simulink model "dqpsk_plot"  (Simulink 4.00)
settings: Solver=ode45  StartTime=0.0  StopTime=10.0  RelTol=1e-3
undefined symbols (not defined in the file): slcm
libraries: commdigbbndpm2 x1, commsource2 x1, simulink3 x1
settings Model: LastModifiedBy=agaltman  BlockReductionOpt=off

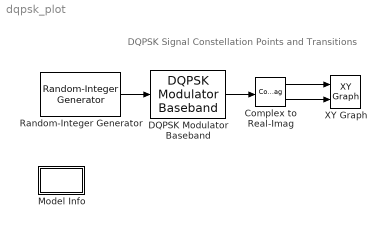
== system dqpsk_plot ==
  note: DQPSK Signal Constellation Points and Transitions
  Complex to Real-Imag : ComplexToRealImag  Output=RealAndImag
  DQPSK Modulator Baseband : commdigbbndpm2/DQPSK Modulator Baseband  InType=Integer  Enc=Binary  Ph=pi/4  numSamp=1
  Model Info : Subsystem  LoadFcn=slcm LoadBlock;  InitFcn=slcm('UpdateAllCMBlocksInThisModelInit')  mask(CMBlock){InitialSaveTempField=, InitialBlockCM=none, BlockCM=none, Frame=on, SaveTempField=, DisplayStringWithTags=Info, MaskDisplayString=Info, HorizontalTextAlignment=Center, LeftAlignmentValue=0.5, SourceBlockDiagram=dqpsk_plot, TagMaxNumber=20, CMTag1=, CMTag2=, CMTag3=, CMTag4=, CMTag5=, CMTag6=, CMTag7=, CMTag8=, CMTag9=, CMTag10=, CMTag11=, CMTag12=, CMTag13=, CMTag14=, CMTag15=, CMTag16=, CMTag17=, CMTag18=, CMTag19=, CMTag20=}
      mask help: This block allows revision control information to be displayed within the model.
      settings: CopyFcn=slcm CopyBlock;  DeleteFcn=slcm Cancel;  PostSaveFcn=slcm('UpdateAllCMBlocksInThisModel')  NameChangeFcn=slcm Rename;  OpenFcn=commdemohelp;  RTWFcnNameOpts=Auto  RTWFileNameOpts=Auto
      mask Display: text(str2num(LeftAlignmentValue), 0.5, MaskDisplayString, 'HorizontalAlignment', HorizontalTextAlignment)
  Random-Integer Generator : commsource2/Random-Integer Generator  mul=4  seed=12345  Ts=.01  frameBased=off  sampPerFrame=1  orient=off
  XY Graph : simulink3/Sinks/XY Graph  xmin=-1  xmax=1  ymin=-1  ymax=1  st=-1
  wires:
  Random-Integer Generator/1 -> DQPSK Modulator Baseband/1
  DQPSK Modulator Baseband/1 -> Complex to Real-Imag/1
  Complex to Real-Imag/1 -> XY Graph/1
  Complex to Real-Imag/2 -> XY Graph/2

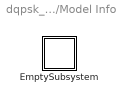
== system dqpsk_plot/Model Info ==
  EmptySubsystem : Subsystem
      settings: RTWFcnNameOpts=Auto  RTWFileNameOpts=Auto

== system dqpsk_plot/Model Info/EmptySubsystem ==
